simulink model "pelican_sim"  (Simulink 7.6)
settings: Solver=ode45  StartTime=0.0  StopTime=1.5  RelTol=1e-3
values from neighbouring files (symbols this model uses):
  xyd = str2double( answer )    [main.m]
libraries: simulink x1
settings Model: Creator=rj  LastModifiedBy=rj
settings DataIOCC: InitialState=q0  LoadInitialState=on

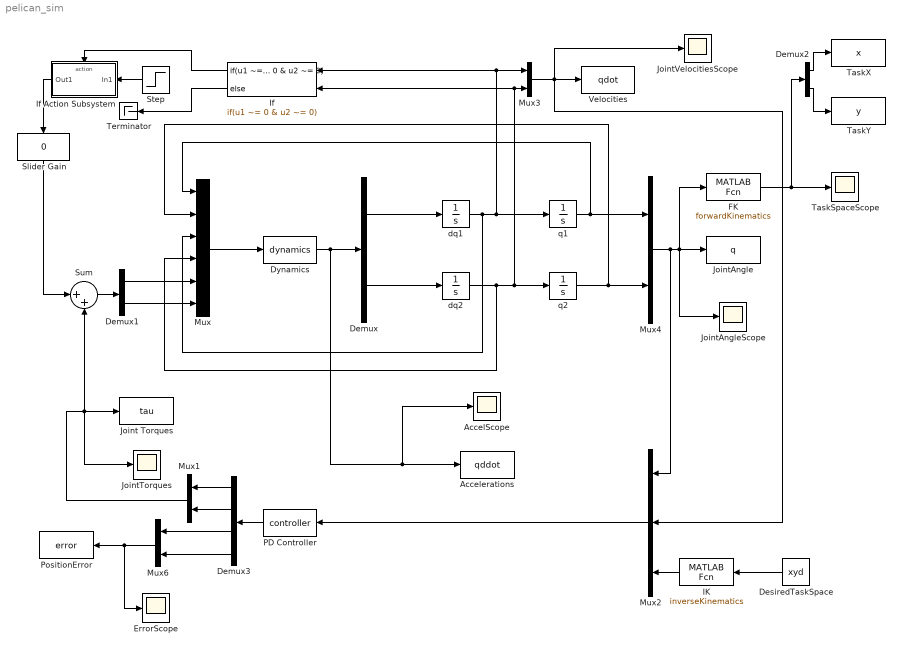
== system pelican_sim ==
  AccelScope : Scope
      settings: YMin=-1e+10  YMax=1e+10  SaveName=AccelScopeData  DataFormat=Array
  Accelerations : ToWorkspace  VariableName=qddot  SampleTime=-1  SaveFormat=Structure
  Demux : Demux  Tag=Demux  Outputs=2
  Demux1 : Demux  Outputs=2
  Demux2 : Demux  Outputs=2
  Demux3 : Demux
  DesiredTaskSpace : Constant  Value=xyd  VectorParams1D=off
  Dynamics : MATLABFcn  MATLABFcn=dynamics  OutputDimensions=2  Output1D=off
  ErrorScope : Scope
      settings: SaveName=ErrorScopeData  DataFormat=Array
  FK : MATLABFcn  MATLABFcn=forwardKinematics  OutputDimensions=2
  IK : MATLABFcn  MATLABFcn=inverseKinematics  OutputDimensions=2  Output1D=off
  If : If  NumInputs=2  IfExpression=u1 ~= 0 & u2 ~= 0
  If Action Subsystem : Subsystem  TreatAsAtomicUnit=on
  Joint Torques : ToWorkspace  VariableName=tau  SampleTime=-1  SaveFormat=Structure
  JointAngle : ToWorkspace  VariableName=q  SampleTime=-1  SaveFormat=Array
  JointAngleScope : Scope
      settings: YMin=-37500  YMax=2500  SaveName=JointAngleScopeData  DataFormat=Array
  JointTorques : Scope
      settings: SaveName=JointTorqScopeData  DataFormat=Array
  JointVelocitiesScope : Scope
      settings: TimeRange=1.5  YMin=-40000  YMax=2500  SaveName=JointVelocitiesScopeData  DataFormat=Array
  Mux : Mux  Inputs=6
  Mux{1,3..4,6} (4 alike) : Mux  Inputs=2
  Mux2 : Mux  Inputs=3
  PD Controller : MATLABFcn  MATLABFcn=controller  OutputDimensions=4  Output1D=off
  PositionError : ToWorkspace  VariableName=error  SampleTime=-1  SaveFormat=Structure
  Slider Gain : simulink/Math Operations/Slider Gain  SystemSampleTime=-1  low=0  gain=0  high=2
  Step : Step  SampleTime=0
  Sum : Sum  Inputs=|++
  TaskSpaceScope : Scope
      settings: TickLabels=on  SaveName=TaskSpaceScopeData  DataFormat=Array
  TaskX : ToWorkspace  VariableName=x  SampleTime=-1  SaveFormat=Array
  TaskY : ToWorkspace  VariableName=y  SampleTime=-1  SaveFormat=Array
  Terminator : Terminator
  Velocities : ToWorkspace  VariableName=qdot  SampleTime=-1  SaveFormat=Structure
  dq1 : Integrator
  dq2 : Integrator
  q1 : Integrator
  q2 : Integrator
  wires:
  Mux/1 -> Dynamics/1
  Dynamics/1 -> Demux/1, Accelerations/1, AccelScope/1
  Demux/1 -> dq1/1
  Demux/2 -> dq2/1
  Demux1/1 -> Mux/5
  Demux1/2 -> Mux/6
  Mux3/1 -> Velocities/1, Mux2/2, JointVelocitiesScope/1
  dq2/1 -> Mux/4, q2/1, Mux3/2, If/2
  dq1/1 -> Mux/3, q1/1, Mux3/1, If/1
  q1/1 -> Mux4/1, Mux/1
  q2/1 -> Mux4/2, Mux/2
  Mux4/1 -> JointAngle/1, JointAngleScope/1, FK/1, Mux2/1
  Mux2/1 -> PD Controller/1
  DesiredTaskSpace/1 -> IK/1
  IK/1 -> Mux2/3
  FK/1 -> TaskSpaceScope/1, Demux2/1
  Demux2/1 -> TaskX/1
  Demux2/2 -> TaskY/1
  PD Controller/1 -> Demux3/1
  Demux3/1 -> Mux1/1
  Demux3/2 -> Mux1/2
  Mux1/1 -> Sum/2, Joint Torques/1, JointTorques/1
  Demux3/3 -> Mux6/1
  Demux3/4 -> Mux6/2
  Mux6/1 -> PositionError/1, ErrorScope/1
  Sum/1 -> Demux1/1
  If/2 -> Terminator/1
  Slider Gain/1 -> Sum/1
  If/1 -> If Action Subsystem/Action
  If Action Subsystem/1(Out1) -> Slider Gain/1
  Step/1 -> If Action Subsystem/1(In1)

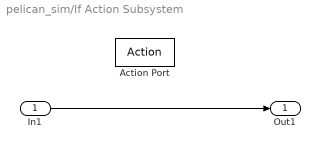
== system pelican_sim/If Action Subsystem ==
  In1 : Inport
  Action Port : ActionPort  ActionType=then
  Out1 : Outport
  wires:
  In1/1 -> Out1/1
